simulink model "P1_Simulink"  (R2024b)
settings: Solver=VariableStepAuto  StartTime=0.0  StopTime=12  RelTol=1e-3
undefined symbols (not defined in the file): DiscIntNeverNeededParam
libraries: SignalEditorBlockLib x1
settings Model: Creator=Usuario_UMA  LastModifiedBy=Mountain
settings RTWCC: GPUComputeCapability=3.5

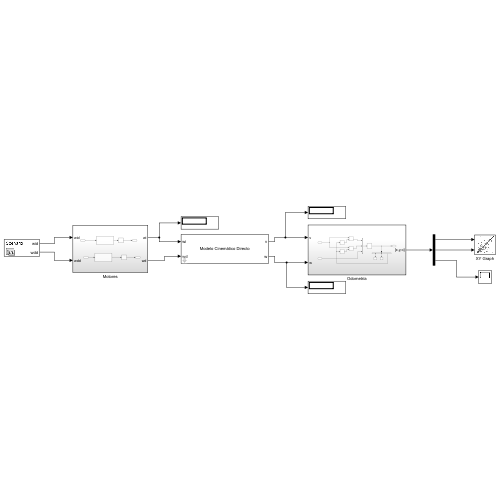
[thumbnail: Simulink's stored preview of the top-level diagram]
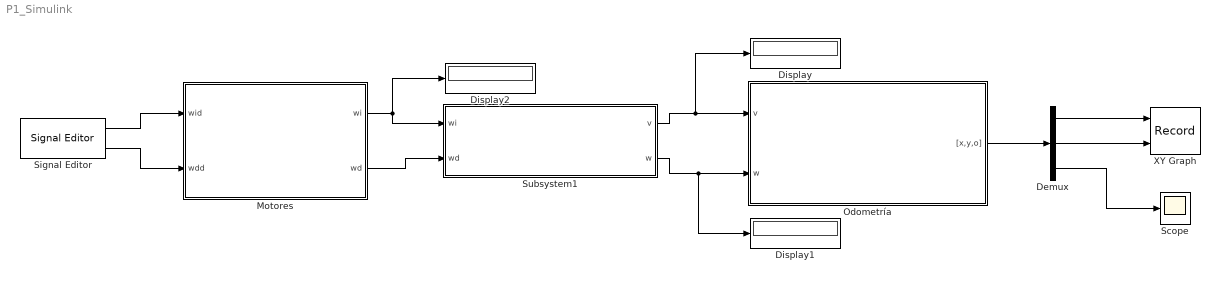
== system P1_Simulink ==
  Demux : Demux  Outputs=3
  Display : Display
  Display1 : Display
  Display2 : Display
  Motores : Subsystem
  Odometría : Subsystem
  Scope : Scope
  Signal Editor : SignalEditorBlockLib/Signal Editor  FileName=trayectoria.mat  ActiveScenario=Scenario  ActiveSignal=wid  IsBus=off  OutputBusObjectStr=Bus: BusObject  SampleTime=0  Interpolate=off  ZeroCross=off  OutputAfterFinalValue=Setting to zero  Unit=inherit  PreserveSignalName=on  ApplySigPropsToAllScenarios=on  ApplySigPropsToAllSignals=off
  Subsystem1 : Subsystem  mask{R=0.1, K=0.4}
      mask prompts: R "Radio de las ruedas"; K "Distancia de la rueda al centro del robot"
      mask Display:
      | disp('Modelo Cinemático Directo');
      | port_label('output', 1, 'v');
      | port_label('output', 2, 'w');
      | port_label('input', 1, 'wi');
      | port_label('input', 2, 'wd');
  XY Graph : Record  FileSettingsInternal="{\"entries\":[{\"content\":{\"excelSettings\":{\"content\":{},\"type\":\"Streamout.ExcelSettings\"}},\"type\":\"Streamout.FileSettingStorage\",\"uuid\":\"\"}],\"packageUris\":[\"http:\\/\\/schema.mathworks.com\\/mf0\\/streamout_blocks\\/R2020a\"],\"version\":\"1.0\"}"  Layout=[1 1]  SignalsInternal="{\"entries\":[{\"content\":{\"signals\":[{\"content\":{\"blockPath\":[],\"dimensions\":[1],\"domain\":\"\",\"lineColor\":\"#a2142f\",\"plots\":[ 1 ],\"port\":1,\"signalID\":1,\"signalName\":\"Demux:1\"},\"type\":\"RecordBlkView.Signal\",\"uuid\":\"\"},{\"content\":{\"blockPath\":[],\"dimensions\":[1],\"domain\":\"\",\"lineColor\":\"#139fff\",\"plots\":[ 1 ],\"port\":2,\"signalID\":2,\"signalName\":\"Demux:2\"},\"type\":\"RecordBlkView.Signal\",\"uuid\":\"\"}]},\"type\":\"RecordBlkView.InputSignals\",\"uuid\":\"\"}],\"packageUris\":[\"http:\\/\\/schema.mathworks.com\\/mf0\\/streamout_blocks\\/R2020a\"],\"version\":\"1.0\"}"  VisualizationBindings="{\"xyplotplugin\":{\"info\":[{\"series\":[{\"bindingParametersList\":[{\"parameter\":\"X-Axis\",\"signalID\":1,\"signalName\":\"Demux:1\"},{\"parameter\":\"Y-Axis\",\"signalID\":2,\"signalName\":\"Demux:2\"}],\"seriesID\":0}],\"subplotID\":1}]}}"  CompatibilityTag=XY
  wires:
  Signal Editor/1 -> Motores/1(wid)
  Signal Editor/2 -> Motores/2(wdd)
  Motores/1(wi) -> Display2/1, Subsystem1/1(wi)
  Motores/2(wd) -> Subsystem1/2(wd)
  Subsystem1/1(v) -> Odometría/1(v), Display/1
  Subsystem1/2(w) -> Display1/1, Odometría/2(w)
  Odometría/1("[x,y,o]") -> Demux/1
  Demux/1 -> XY Graph/1
  Demux/2 -> XY Graph/2
  Demux/3 -> Scope/1

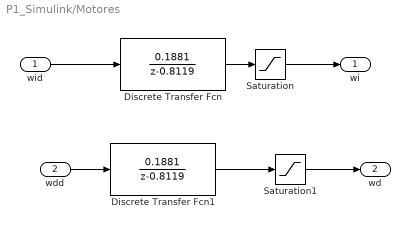
== system P1_Simulink/Motores ==
  wid : Inport
  wdd : Inport  Port=2
  Discrete Transfer Fcn : DiscreteTransferFcn  Numerator=[0.1881]  Denominator=[1 -0.8119]
  Discrete Transfer Fcn1 : DiscreteTransferFcn  Numerator=[0.1881]  Denominator=[1 -0.8119]
  Saturation : Saturate  UpperLimit=15  LowerLimit=-15
  Saturation1 : Saturate  UpperLimit=15  LowerLimit=-15
  wi : Outport
  wd : Outport  Port=2
  wires:
  wid/1 -> Discrete Transfer Fcn/1
  Discrete Transfer Fcn1/1 -> Saturation1/1
  wdd/1 -> Discrete Transfer Fcn1/1
  Saturation/1 -> wi/1
  Saturation1/1 -> wd/1
  Discrete Transfer Fcn/1 -> Saturation/1

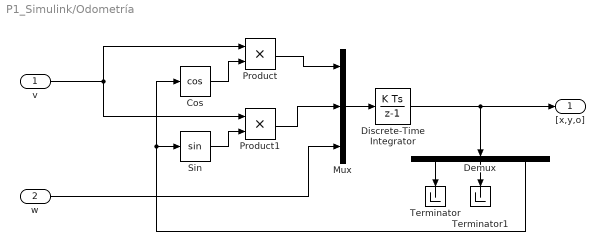
== system P1_Simulink/Odometría ==
  v : Inport
  w : Inport  Port=2
  Cos : Trigonometry  Operator=cos
  Demux : Demux  Outputs=3
  Discrete-Time Integrator : DiscreteIntegrator  SampleTime=0.025  ICPrevOutput=DiscIntNeverNeededParam  ICPrevScaledInput=DiscIntNeverNeededParam
  Mux : Mux  Inputs=3
  Product : Product
  Product1 : Product
  Sin : Trigonometry
  Terminator : Terminator
  Terminator1 : Terminator
  "[x,y,o]" : Outport
  wires:
  Cos/1 -> Product/2
  Product/1 -> Mux/1
  Demux/3 -> Cos/1, Sin/1
  Demux/1 -> Terminator/1
  Product1/1 -> Mux/2
  Demux/2 -> Terminator1/1
  Sin/1 -> Product1/2
  w/1 -> Mux/3
  Mux/1 -> Discrete-Time Integrator/1
  v/1 -> Product1/1, Product/1
  Discrete-Time Integrator/1 -> "[x,y,o]"/1, Demux/1

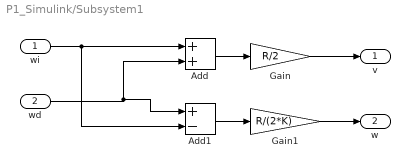
== system P1_Simulink/Subsystem1 ==
  wi : Inport
  wd : Inport  Port=2
  Add : Sum
  Add1 : Sum  Inputs=+-
  Gain : Gain  Gain=R/2
  Gain1 : Gain  Gain=R/(2*K)
  v : Outport
  w : Outport  Port=2
  wires:
  Add/1 -> Gain/1
  wi/1 -> Add1/2, Add/1
  wd/1 -> Add1/1, Add/2
  Gain/1 -> v/1
  Add1/1 -> Gain1/1
  Gain1/1 -> w/1
